simulink model "ptp_and_time_sharing"  (R2024b)
settings: Solver=ode1be  StartTime=0.0  StopTime=40e-3  FixedStep=ts  RelTol=1e-3
undefined symbols (not defined in the file): time_gain_1, time_gain_2, ts_ctrl
libraries: spsSampleandHoldLib x2
settings Model: Creator=ltnbda  LastModifiedBy=ltnbda

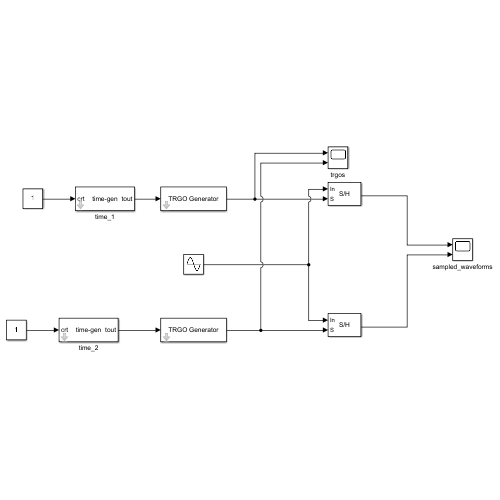
[thumbnail: Simulink's stored preview of the top-level diagram]
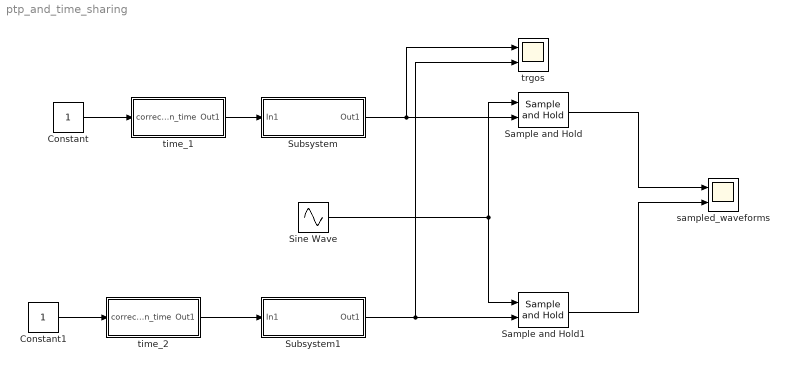
== system ptp_and_time_sharing ==
  Constant : Constant
  Constant1 : Constant
  Sample and Hold : spsSampleandHoldLib/Sample and Hold  ic=0  Ts=0
      settings: LibrarySourceBlock=|
      | sps_lib/Control/Sample and
      | Hold
  Sample and Hold1 : spsSampleandHoldLib/Sample and Hold  ic=0  Ts=0
      settings: LibrarySourceBlock=|
      | sps_lib/Control/Sample and
      | Hold
  Sine Wave : Sin  Frequency=50*2*pi  SampleTime=0
  Subsystem : Subsystem  mask{samplig_time=ts_ctrl}
      mask prompts: samplig_time "Sampling Time"
      mask Display: disp('TRGO Generator');
  Subsystem1 : Subsystem  mask{samplig_time=ts_ctrl}
      mask prompts: samplig_time "Sampling Time"
      mask Display: disp('TRGO Generator');
  sampled_waveforms : Scope  NumInputPorts=2
  time_1 : Subsystem  mask{k=time_gain_1}
      mask prompts: k "Time Gain"
      mask Display:
      | disp('time-gen');
      | port_label('input', 1, 'crt');
      | port_label('output', 1, 'tout');
  time_2 : Subsystem  mask{k=time_gain_2}
      mask prompts: k "Time Gain"
      mask Display:
      | disp('time-gen');
      | port_label('input', 1, 'crt');
      | port_label('output', 1, 'tout');
  trgos : Scope  NumInputPorts=2
  wires:
  Sine Wave/1 -> Sample and Hold/1, Sample and Hold1/1
  Sample and Hold/1 -> sampled_waveforms/1
  Sample and Hold1/1 -> sampled_waveforms/2
  Subsystem1/1(Out1) -> trgos/2, Sample and Hold1/2
  Subsystem/1(Out1) -> Sample and Hold/2, trgos/1
  time_1/1(Out1) -> Subsystem/1(In1)
  time_2/1(Out1) -> Subsystem1/1(In1)
  Constant/1 -> time_1/1(correction_time)
  Constant1/1 -> time_2/1(correction_time)

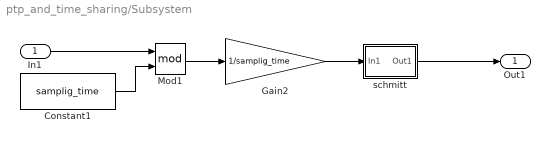
== system ptp_and_time_sharing/Subsystem ==
  In1 : Inport
  Constant1 : Constant  Value=samplig_time
  Gain2 : Gain  Gain=1/samplig_time
  Mod1 : Math  Operator=mod
  schmitt : Subsystem
  Out1 : Outport
  wires:
  Constant1/1 -> Mod1/2
  In1/1 -> Mod1/1
  Mod1/1 -> Gain2/1
  schmitt/1(Out1) -> Out1/1
  Gain2/1 -> schmitt/1(In1)

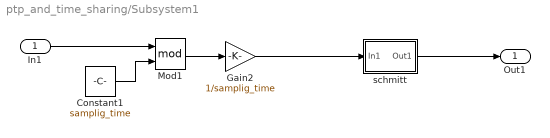
== system ptp_and_time_sharing/Subsystem1 ==
  In1 : Inport
  Constant1 : Constant  Value=samplig_time
  Gain2 : Gain  Gain=1/samplig_time
  Mod1 : Math  Operator=mod
  schmitt : Subsystem
  Out1 : Outport
  wires:
  Gain2/1 -> schmitt/1(In1)
  schmitt/1(Out1) -> Out1/1
  Mod1/1 -> Gain2/1
  In1/1 -> Mod1/1
  Constant1/1 -> Mod1/2

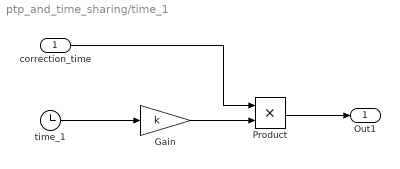
== system ptp_and_time_sharing/time_1 ==
  correction_time : Inport
  Gain : Gain  Gain=k
  Product : Product
  time_1 : Clock
  Out1 : Outport
  wires:
  time_1/1 -> Gain/1
  Gain/1 -> Product/2
  Product/1 -> Out1/1
  correction_time/1 -> Product/1

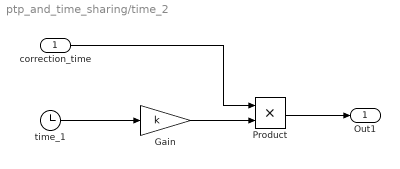
== system ptp_and_time_sharing/time_2 ==
  correction_time : Inport
  Gain : Gain  Gain=k
  Product : Product
  time_1 : Clock
  Out1 : Outport
  wires:
  correction_time/1 -> Product/1
  Product/1 -> Out1/1
  Gain/1 -> Product/2
  time_1/1 -> Gain/1

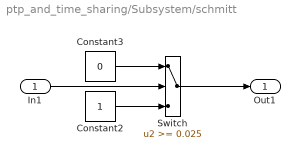
== system ptp_and_time_sharing/Subsystem/schmitt ==
  In1 : Inport
  Constant2 : Constant
  Constant3 : Constant  Value=0
  Switch : Switch  Threshold=0.025  SaturateOnIntegerOverflow=off  InputSameDT=off
  Out1 : Outport
  wires:
  Constant2/1 -> Switch/3
  Constant3/1 -> Switch/1
  In1/1 -> Switch/2
  Switch/1 -> Out1/1

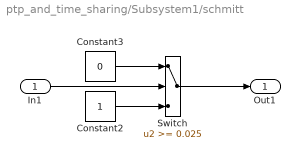
== system ptp_and_time_sharing/Subsystem1/schmitt ==
  In1 : Inport
  Constant2 : Constant
  Constant3 : Constant  Value=0
  Switch : Switch  Threshold=0.025  SaturateOnIntegerOverflow=off  InputSameDT=off
  Out1 : Outport
  wires:
  Switch/1 -> Out1/1
  In1/1 -> Switch/2
  Constant3/1 -> Switch/1
  Constant2/1 -> Switch/3
